simulink model "Selector_TestGen20"  (R2017b)
settings: Solver=FixedStepDiscrete  StartTime=0.0  StopTime=10.0  RelTol=1e-3
settings Model: Creator=ktrinh  LastModifiedBy=ktrinh
settings DebuggingCC: ParameterOverflowMsg=none

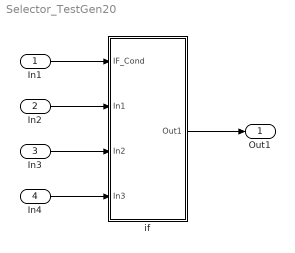
== system Selector_TestGen20 ==
  In1 : Inport
  In2 : Inport  Port=2
  In3 : Inport  Port=3
  In4 : Inport  Port=4
  if : Subsystem  AncestorBlock=Block_TestLib/if
  Out1 : Outport
  wires:
  In1/1 -> if/1(IF_Cond)
  In2/1 -> if/2(In1)
  In3/1 -> if/3(In2)
  In4/1 -> if/4(In3)
  if/1(Out1) -> Out1/1

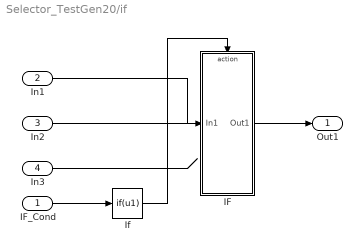
== system Selector_TestGen20/if ==
  IF_Cond : Inport  OutDataTypeStr=boolean
  In1 : Inport  Port=2
  In2 : Inport  Port=3
  In3 : Inport  Port=4
  IF : Subsystem  TreatAsAtomicUnit=on
  If : If  IfExpression=u1  ShowElse=off
  Out1 : Outport
  wires:
  If/1 -> IF/Action
  In1/1 -> IF/1(In1)
  In2/1 -> ?
  In3/1 -> ?
  IF_Cond/1 -> If/1
  IF/1(Out1) -> Out1/1

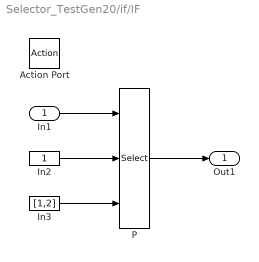
== system Selector_TestGen20/if/IF ==
  In1 : Inport  OutDataTypeStr=double  PortDimensions=[2 3 2 2]
  Action Port : ActionPort  ActionType=then
  In2 : Constant
  In3 : Constant  Value=[1,2]
  P : Selector  NumberOfDimensions=4  InputPortWidth=3  IndexOptions=Starting index (port),Select all,Index vector (dialog),Index vector (port)  Indices=[],[],[1,2],[]  OutputSizes=2,,,
  Out1 : Outport
  wires:
  In1/1 -> P/1
  In2/1 -> P/2
  In3/1 -> P/3
  P/1 -> Out1/1
